simulink model "Simulator"  (R2020a)
settings: Solver=FixedStepAuto  StartTime=0.0  StopTime=10.0  FixedStep=0.02  RelTol=1e-3
values from neighbouring files (symbols this model uses):
  g = data(5); Quad.b = data(6); Quad.d = data(7); Quad.l = data(8)    [Quad1.m]
undefined symbols (not defined in the file or in its folder): Quad
libraries: shared6dof x1
settings Model: Creator=Hisham  LastModifiedBy=Hisham
settings DataIOCC: ReturnWorkspaceOutputs=off
settings DebuggingCC: ArithmeticOperatorsInVariantConditions=warning
settings SFSimCC: SimUseLocalCustomCode=off  CustomCodeUndefinedFunction=UseInterfaceOnly
settings RTWCC: RTWUseLocalCustomCode=off
settings CodeAppCC: StateflowObjectComments=on

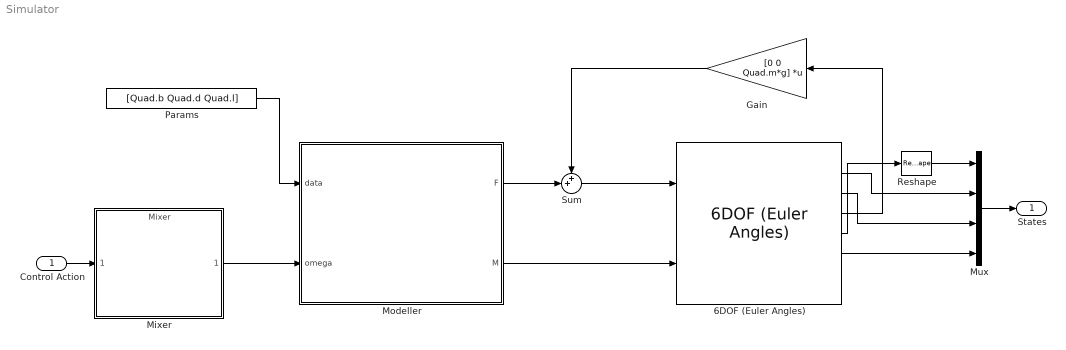
== system Simulator ==
  Control Action : Inport
  6DOF (Euler Angles) : shared6dof/6DOF (Euler Angles)  units=Metric (MKS)  mtype=Fixed  rep=Euler Angles  xme_0=[0 0 -1]  Vm_0=[0 0 0]  eul_0=[0 0 0]*pi/180  pm_0=[0 0 0]  mass_0=Quad.m  mass_e=0.5  mass_f=2.0  inertia=Quad.I  inertia_e=eye(3)  inertia_f=2*eye(3)  k_quat=1.0  vre_flag=on  abi_flag=off  aMode=aMode  xme_statename=''  Vm_statename=''  eul_statename=''  quat_statename=''  pm_statename=''  mass_statename=''
      settings: SourceProductBaseCode=AE,PW,MT,VE,VP
  Gain : Gain  Gain=[0 0 Quad.m*g]  Multiplication=Matrix(K*u)
  Mixer : ModelReference  ModelNameDialog=Mixer.slx  SimulationMode=Normal  ModelReferenceVersion=1.11
  Modeller : MATLAB Function  TreatAsAtomicUnit=on
  Mux : Mux
  Params : Constant  Value=[Quad.b Quad.d Quad.l]
  Reshape : Reshape  OutputDimensions=3x1
  Sum : Sum  Inputs=++|
  States : Outport
  wires:
  Modeller/2(M) -> 6DOF (Euler Angles)/2
  6DOF (Euler Angles)/4 -> Gain/1
  Gain/1 -> Sum/1
  Modeller/1(F) -> Sum/2
  Sum/1 -> 6DOF (Euler Angles)/1
  6DOF (Euler Angles)/2 -> Mux/2
  Mux/1 -> States/1
  Params/1 -> Modeller/1(data)
  6DOF (Euler Angles)/3 -> Mux/3
  6DOF (Euler Angles)/6 -> Mux/4
  Mixer/1 -> Modeller/2(omega)
  Control Action/1 -> Mixer/1
  6DOF (Euler Angles)/5 -> Reshape/1
  Reshape/1 -> Mux/1

== matlab function Simulator/Modeller ==
  data: data input; omega input; F output; M output
function [F,M] = fcn(data, omega)
b = data(1);
d = data(2);
l = data(3);
F = zeros(1,3); M = F;
F(1) = 0;
F(2) = 0;
F(3) = -b*(omega(1)^2 + omega(2)^2 + omega(3)^2 + omega(4)^2);
M(1) = b*l*(omega(4)^2 - omega(2)^2);
M(2) = b*l*(omega(1)^2 - omega(3)^2);
M(3) = d*(omega(1)^2 + omega(3)^2 - omega(2)^2 - omega(4)^2);
